simulink library "powerlib_extras"  (Simulink 6.0)
settings: Solver=ode45  SolverMode=SingleTasking  StartTime=0.0  StopTime=10.0  RelTol=1e-3
values from neighbouring files (symbols this model uses):
  Ts = get(handles.edit1,'string')    [powergui.m]
undefined symbols (not defined in the file or in its folder): Ac, Bc, Cc, Dc, Delay_discrete, dend, DiscIntNeverNeededParam, extra_sc, j, numd, test_alpha
libraries: powerlib2 x112, powerlib_extras x70, simulink_extras x25, simulink x12, powerlib_models x8
(part 8 of 9)

== system powerlib_extras/Measurements/3-Phase Sequence Analyzer/PhasorA ==
  in : Inport  Port=1  LatchInput=off
  sin : Inport  Port=2  LatchInput=off
  cos : Inport  Port=3  LatchInput=off
  Gain1 : Gain  Gain=k*f1  SaturateOnIntegerOverflow=on
  Integ2 : Integrator
  Product : Product  SaturateOnIntegerOverflow=on  InputSameDT=on
  Product1 : Product  SaturateOnIntegerOverflow=on  InputSameDT=on
  Real-Imag to Complex : RealImagToComplex
  Sum2 : Sum  Inputs=+-  SaturateOnIntegerOverflow=on  InputSameDT=on
  Sum3 : Sum  Inputs=+-  SaturateOnIntegerOverflow=on  InputSameDT=on
  T : TransportDelay  DelayTime=1/f1
  T1 : TransportDelay  DelayTime=1/f1
  integ1 : Integrator
  Out : Outport  InitialOutput=0
  wires:
  Real-Imag to Complex/1 -> Out/1
  Sum3/1 -> Real-Imag to Complex/2
  Sum2/1 -> Real-Imag to Complex/1
  Product/1 -> integ1/1
  Product1/1 -> Integ2/1
  T/1 -> Sum2/2
  T1/1 -> Sum3/2
  integ1/1 -> T/1, Sum2/1
  Integ2/1 -> T1/1, Sum3/1
  Gain1/1 -> Product1/1, Product/2
  sin/1 -> Product/1
  in/1 -> Gain1/1
  cos/1 -> Product1/2

== system powerlib_extras/Measurements/3-Phase Sequence Analyzer/PhasorB ==
  in : Inport  Port=1  LatchInput=off
  sin : Inport  Port=2  LatchInput=off
  cos : Inport  Port=3  LatchInput=off
  Gain1 : Gain  Gain=k*f1  SaturateOnIntegerOverflow=on
  Integ2 : Integrator
  Product : Product  SaturateOnIntegerOverflow=on  InputSameDT=on
  Product1 : Product  SaturateOnIntegerOverflow=on  InputSameDT=on
  Real-Imag to Complex : RealImagToComplex
  Sum2 : Sum  Inputs=+-  SaturateOnIntegerOverflow=on  InputSameDT=on
  Sum3 : Sum  Inputs=+-  SaturateOnIntegerOverflow=on  InputSameDT=on
  T : TransportDelay  DelayTime=1/f1
  T1 : TransportDelay  DelayTime=1/f1
  integ1 : Integrator
  Out : Outport  InitialOutput=0
  wires:
  cos/1 -> Product1/2
  in/1 -> Gain1/1
  sin/1 -> Product/1
  Gain1/1 -> Product/2, Product1/1
  Integ2/1 -> Sum3/1, T1/1
  integ1/1 -> Sum2/1, T/1
  T1/1 -> Sum3/2
  T/1 -> Sum2/2
  Product1/1 -> Integ2/1
  Product/1 -> integ1/1
  Sum2/1 -> Real-Imag to Complex/1
  Sum3/1 -> Real-Imag to Complex/2
  Real-Imag to Complex/1 -> Out/1

== system powerlib_extras/Measurements/3-Phase Sequence Analyzer/PhasorC ==
  in : Inport  Port=1  LatchInput=off
  sin : Inport  Port=2  LatchInput=off
  cos : Inport  Port=3  LatchInput=off
  Gain1 : Gain  Gain=k*f1  SaturateOnIntegerOverflow=on
  Integ2 : Integrator
  Product : Product  SaturateOnIntegerOverflow=on  InputSameDT=on
  Product1 : Product  SaturateOnIntegerOverflow=on  InputSameDT=on
  Real-Imag to Complex : RealImagToComplex
  Sum2 : Sum  Inputs=+-  SaturateOnIntegerOverflow=on  InputSameDT=on
  Sum3 : Sum  Inputs=+-  SaturateOnIntegerOverflow=on  InputSameDT=on
  T : TransportDelay  DelayTime=1/f1
  T1 : TransportDelay  DelayTime=1/f1
  integ1 : Integrator
  Out : Outport  InitialOutput=0
  wires:
  Real-Imag to Complex/1 -> Out/1
  Sum3/1 -> Real-Imag to Complex/2
  Sum2/1 -> Real-Imag to Complex/1
  Product/1 -> integ1/1
  Product1/1 -> Integ2/1
  T/1 -> Sum2/2
  T1/1 -> Sum3/2
  integ1/1 -> T/1, Sum2/1
  Integ2/1 -> T1/1, Sum3/1
  Gain1/1 -> Product1/1, Product/2
  sin/1 -> Product/1
  in/1 -> Gain1/1
  cos/1 -> Product1/2

== system powerlib_extras/Measurements/3-Phase Sequence Analyzer/Pos. Seq. Computation ==
  In : Inport  Port=1  LatchInput=off
  Enable : EnablePort
  Gain1 : Gain  Gain=[1 a a2]  SaturateOnIntegerOverflow=on
  Gain3 : Gain  Gain=1/3  SaturateOnIntegerOverflow=on
  Sum : Sum  Inputs=1  SaturateOnIntegerOverflow=on  InputSameDT=on
  Out : Outport
  wires:
  Gain1/1 -> Sum/1
  Sum/1 -> Gain3/1
  In/1 -> Gain1/1
  Gain3/1 -> Out/1

== system powerlib_extras/Measurements/3-Phase Sequence Analyzer/Zero Seq. Computation ==
  In : Inport  Port=1  LatchInput=off
  Enable : EnablePort
  Gain3 : Gain  Gain=1/3  SaturateOnIntegerOverflow=on
  Sum : Sum  Inputs=1  SaturateOnIntegerOverflow=on  InputSameDT=on
  Out : Outport
  wires:
  Sum/1 -> Gain3/1
  In/1 -> Sum/1
  Gain3/1 -> Out/1

== system powerlib_extras/Phasor Library/Sequence Analyzer (Phasor Type)/Neg. Seq. Computation ==
  In : Inport  Port=1  LatchInput=off
  Enable : EnablePort
  Gain1 : Gain  Gain=[1 a2 a]  SaturateOnIntegerOverflow=on
  Gain3 : Gain  Gain=1/3  SaturateOnIntegerOverflow=on
  Sum : Sum  Inputs=1  SaturateOnIntegerOverflow=on  InputSameDT=on
  Out : Outport
  wires:
  Gain3/1 -> Out/1
  In/1 -> Gain1/1
  Sum/1 -> Gain3/1
  Gain1/1 -> Sum/1

== system powerlib_extras/Phasor Library/Sequence Analyzer (Phasor Type)/Pos. Seq. Computation ==
  In : Inport  Port=1  LatchInput=off
  Enable : EnablePort
  Gain1 : Gain  Gain=[1 a a2]  SaturateOnIntegerOverflow=on
  Gain3 : Gain  Gain=1/3  SaturateOnIntegerOverflow=on
  Sum : Sum  Inputs=1  SaturateOnIntegerOverflow=on  InputSameDT=on
  Out : Outport
  wires:
  Gain3/1 -> Out/1
  In/1 -> Gain1/1
  Sum/1 -> Gain3/1
  Gain1/1 -> Sum/1

== system powerlib_extras/Phasor Library/Sequence Analyzer (Phasor Type)/Zero Seq. Computation ==
  In : Inport  Port=1  LatchInput=off
  Enable : EnablePort
  Gain3 : Gain  Gain=1/3  SaturateOnIntegerOverflow=on
  Sum : Sum  Inputs=1  SaturateOnIntegerOverflow=on  InputSameDT=on
  Out : Outport
  wires:
  Gain3/1 -> Out/1
  In/1 -> Sum/1
  Sum/1 -> Gain3/1

== system powerlib_extras/Phasor Library/Static Var Compensator (Phasor Type)/Currrent phasor ==
  I1 : Inport  Port=1  LatchInput=off
  I2 : Inport  Port=2  LatchInput=off
  Mux1 : Mux  Inputs=2
  Sum1 : Sum  SaturateOnIntegerOverflow=on  InputSameDT=on
  Sum3 : Sum  SaturateOnIntegerOverflow=on  InputSameDT=on
  a : Gain  Gain=exp(j*2*pi/3)  SaturateOnIntegerOverflow=on
  a^2 : Gain  Gain=exp(-j*2*pi/3)  SaturateOnIntegerOverflow=on
  Ia Ib cmplx : Outport
  wires:
  Mux1/1 -> Ia Ib cmplx/1  "ia ib"
  Sum1/1 -> Mux1/2
  Sum3/1 -> Mux1/1
  a/1 -> Sum1/2
  a^2/1 -> Sum1/1
  I2/1 -> Sum3/2, a/1
  I1/1 -> Sum3/1, a^2/1

== system powerlib_extras/Phasor Library/Static Var Compensator (Phasor Type)/I1 Time delay  Td ==
  I1 cmplx : Inport  Orientation=left  Port=1  LatchInput=off
  Complex to Real-Imag : ComplexToRealImag  Orientation=left
  Real-Imag to Complex : RealImagToComplex  Orientation=left
  Transport Delay1 : TransportDelay  Orientation=left  DelayTime=Td
  Transport Delay2 : TransportDelay  Orientation=left  DelayTime=Td
  Out1 : Outport  Orientation=left
  wires:
  I1 cmplx/1 -> Complex to Real-Imag/1
  Real-Imag to Complex/1 -> Out1/1
  Complex to Real-Imag/1 -> Transport Delay1/1
  Complex to Real-Imag/2 -> Transport Delay2/1
  Transport Delay1/1 -> Real-Imag to Complex/1
  Transport Delay2/1 -> Real-Imag to Complex/2

== system powerlib_extras/Phasor Library/Static Var Compensator (Phasor Type)/I2 Time delay I2 ==
  I1 cmplx : Inport  Orientation=left  Port=1  LatchInput=off
  Complex to Real-Imag : ComplexToRealImag  Orientation=left
  Real-Imag to Complex : RealImagToComplex  Orientation=left
  Transport Delay1 : TransportDelay  Orientation=left  DelayTime=Td
  Transport Delay2 : TransportDelay  Orientation=left  DelayTime=Td
  Out1 : Outport  Orientation=left
  wires:
  Transport Delay2/1 -> Real-Imag to Complex/2
  Transport Delay1/1 -> Real-Imag to Complex/1
  Complex to Real-Imag/2 -> Transport Delay2/1
  Complex to Real-Imag/1 -> Transport Delay1/1
  Real-Imag to Complex/1 -> Out1/1
  I1 cmplx/1 -> Complex to Real-Imag/1

== system powerlib_extras/Phasor Library/Static Var Compensator (Phasor Type)/V1 V2 ==
  Vab Vbc cmplx : Inport  Port=1  LatchInput=off
  (a^2)/3 : Gain  Gain=1/3*exp(-j*2*pi/3)  SaturateOnIntegerOverflow=on
  Demux : Demux  Outputs=2
  Gain : Gain  Gain=1/3  SaturateOnIntegerOverflow=on
  Gain1 : Gain  Gain=1/3  SaturateOnIntegerOverflow=on
  Sum3 : Sum  Inputs=+-  SaturateOnIntegerOverflow=on  InputSameDT=on
  Sum4 : Sum  Inputs=+-  SaturateOnIntegerOverflow=on  InputSameDT=on
  V>pu : Gain  Gain=1/Vbase  SaturateOnIntegerOverflow=on
  a/3 : Gain  Gain=1/3*exp(j*2*pi/3)  SaturateOnIntegerOverflow=on
  V1_pu : Outport
  V2_pu : Outport  Port=2
  wires:
  Sum4/1 -> V2_pu/1  "V2"
  (a^2)/3/1 -> Sum3/2
  Demux/2 -> (a^2)/3/1, a/3/1
  Gain/1 -> Sum3/1
  Vab Vbc cmplx/1 -> V>pu/1
  Gain1/1 -> Sum4/1
  a/3/1 -> Sum4/2
  Demux/1 -> Gain/1, Gain1/1
  Sum3/1 -> V1_pu/1  "V1"
  V>pu/1 -> Demux/1

== system powerlib_extras/Phasor Library/Static Var Compensator (Phasor Type)/Voltage regulator ==
  V1meas (pu) : Inport  Port=1  LatchInput=off
  Vref (pu) : Inport  Port=2  LatchInput=off
  Break algebraic loop : TransferFcn  Orientation=left  Denominator=[100e-6 1]
  Droop : Gain  Orientation=left  Gain=Xs  SaturateOnIntegerOverflow=on
  Integrator : Integrator  LimitOutput=on  UpperSaturationLimit=1  LowerSaturationLimit=-1
  Ki : Gain  Gain=Ki  SaturateOnIntegerOverflow=on
  Product : Product  Orientation=down  SaturateOnIntegerOverflow=on  InputSameDT=on
  Sum : Sum  Inputs=-+-  SaturateOnIntegerOverflow=on  InputSameDT=on
  B (pu) : Outport  InitialOutput=0
  wires:
  Product/1 -> Break algebraic loop/1
  Integrator/1 -> B (pu)/1, Product/2
  Sum/1 -> Ki/1
  Vref (pu)/1 -> Sum/2
  Ki/1 -> Integrator/1
  V1meas (pu)/1 -> Sum/1, Product/1
  Droop/1 -> Sum/3
  Break algebraic loop/1 -> Droop/1

== system powerlib_extras/Control  Blocks/ Synchronized 12-Pulse Generator/12 Flip-Flops/6 Flip-Flop ==
  S : Inport  Port=1  LatchInput=off
  R : Inport  Port=2  LatchInput=off
  Demux : Demux  Outputs=6
  Demux1 : Demux  Outputs=6
  Mux : Mux  Inputs=6
  S-R Flip-Flop{1..6} (6 alike) : simulink_extras/Flip Flops/S-R Flip-Flop  initial_condition=0
  Terminator{,1..5} (6 alike) : Terminator
  Q : Outport
  wires:
  S-R Flip-Flop6/2 -> Terminator5/1
  S-R Flip-Flop5/2 -> Terminator4/1
  S-R Flip-Flop4/2 -> Terminator3/1
  S-R Flip-Flop3/2 -> Terminator2/1
  S-R Flip-Flop2/2 -> Terminator1/1
  S-R Flip-Flop1/1 -> Mux/1
  S-R Flip-Flop2/1 -> Mux/2
  S-R Flip-Flop3/1 -> Mux/3
  S-R Flip-Flop4/1 -> Mux/4
  S-R Flip-Flop5/1 -> Mux/5
  Mux/1 -> Q/1
  S-R Flip-Flop6/1 -> Mux/6
  S-R Flip-Flop1/2 -> Terminator/1
  Demux/1 -> S-R Flip-Flop1/1
  Demux/2 -> S-R Flip-Flop2/1
  Demux/3 -> S-R Flip-Flop3/1
  Demux/4 -> S-R Flip-Flop4/1
  S/1 -> Demux/1
  Demux/6 -> S-R Flip-Flop6/1
  Demux/5 -> S-R Flip-Flop5/1
  R/1 -> Demux1/1
  Demux1/1 -> S-R Flip-Flop1/2
  Demux1/2 -> S-R Flip-Flop2/2
  Demux1/3 -> S-R Flip-Flop3/2
  Demux1/4 -> S-R Flip-Flop4/2
  Demux1/5 -> S-R Flip-Flop5/2
  Demux1/6 -> S-R Flip-Flop6/2

== system powerlib_extras/Control  Blocks/ Synchronized 12-Pulse Generator/12 Flip-Flops/6 Flip-Flop1 ==
  S : Inport  Port=1  LatchInput=off
  R : Inport  Port=2  LatchInput=off
  Demux : Demux  Outputs=6
  Demux1 : Demux  Outputs=6
  Mux : Mux  Inputs=6
  S-R Flip-Flop{1..6} (6 alike) : simulink_extras/Flip Flops/S-R Flip-Flop  initial_condition=0
  Terminator{,1..5} (6 alike) : Terminator
  Q : Outport
  wires:
  Demux1/6 -> S-R Flip-Flop6/2
  Demux1/5 -> S-R Flip-Flop5/2
  Demux1/4 -> S-R Flip-Flop4/2
  Demux1/3 -> S-R Flip-Flop3/2
  Demux1/2 -> S-R Flip-Flop2/2
  Demux1/1 -> S-R Flip-Flop1/2
  R/1 -> Demux1/1
  Demux/5 -> S-R Flip-Flop5/1
  Demux/6 -> S-R Flip-Flop6/1
  S/1 -> Demux/1
  Demux/4 -> S-R Flip-Flop4/1
  Demux/3 -> S-R Flip-Flop3/1
  Demux/2 -> S-R Flip-Flop2/1
  Demux/1 -> S-R Flip-Flop1/1
  S-R Flip-Flop1/2 -> Terminator/1
  S-R Flip-Flop6/1 -> Mux/6
  Mux/1 -> Q/1
  S-R Flip-Flop5/1 -> Mux/5
  S-R Flip-Flop4/1 -> Mux/4
  S-R Flip-Flop3/1 -> Mux/3
  S-R Flip-Flop2/1 -> Mux/2
  S-R Flip-Flop1/1 -> Mux/1
  S-R Flip-Flop2/2 -> Terminator1/1
  S-R Flip-Flop3/2 -> Terminator2/1
  S-R Flip-Flop4/2 -> Terminator3/1
  S-R Flip-Flop5/2 -> Terminator4/1
  S-R Flip-Flop6/2 -> Terminator5/1

== system powerlib_extras/Control  Blocks/Monostable/Edge Detector/NEGATIVE Edge ==
  IN : Inport  Port=1  LatchInput=off
  IN previous : Inport  Port=2  LatchInput=off
  Enable : EnablePort
  Relational Operator1 : RelationalOperator  Operator=>  InputSameDT=on
  OUT : Outport
  wires:
  IN/1 -> Relational Operator1/2
  IN previous/1 -> Relational Operator1/1
  Relational Operator1/1 -> OUT/1

== system powerlib_extras/Control  Blocks/Monostable/Edge Detector/POSITIVE Edge ==
  IN : Inport  Port=1  LatchInput=off
  IN previous : Inport  Port=2  LatchInput=off
  Enable : EnablePort
  Relational Operator1 : RelationalOperator  Operator=>  InputSameDT=on
  OUT : Outport
  wires:
  IN/1 -> Relational Operator1/1
  IN previous/1 -> Relational Operator1/2
  Relational Operator1/1 -> OUT/1

== system powerlib_extras/Discrete  Control Blocks/Discrete Monostable/Edge_Detector/NEGATIVE Edge ==
  IN : Inport  Port=1  LatchInput=off
  IN previous : Inport  Port=2  LatchInput=off
  Enable : EnablePort
  Relational Operator1 : RelationalOperator  Operator=>  InputSameDT=on
  OUT : Outport
  wires:
  IN/1 -> Relational Operator1/2
  IN previous/1 -> Relational Operator1/1
  Relational Operator1/1 -> OUT/1

== system powerlib_extras/Discrete  Control Blocks/Discrete Monostable/Edge_Detector/POSITIVE Edge ==
  IN : Inport  Port=1  LatchInput=off
  IN previous : Inport  Port=2  LatchInput=off
  Enable : EnablePort
  Relational Operator1 : RelationalOperator  Operator=>  InputSameDT=on
  OUT : Outport
  wires:
  IN/1 -> Relational Operator1/1
  IN previous/1 -> Relational Operator1/2
  Relational Operator1/1 -> OUT/1

== system powerlib_extras/Discrete  Control Blocks/Discrete 12-Pulse HVDC Control /Functions (Discrete)/Control Mode ==
  note: CONTROL MODE (#):
      |
      | 0) Blocked
      | 1) Current control
      | 2) Voltage control
      | 3) Alpha minimum limitation
      | 4) Alpha maximum limitation
      | 5) Forced or constant Alpha
  "a_ord_i " : Inport  Port=1  LatchInput=off
  a_ord_v : Inport  Port=2  LatchInput=off
  alpha_ord : Inport  Port=3  LatchInput=off
  Max_i : Inport  Port=4  LatchInput=off
  Min_i : Inport  Port=5  LatchInput=off
  Block : Inport  Port=6  LatchInput=off
  C : Constant  Value=0
  Gain1 : Gain  Gain=3  SaturateOnIntegerOverflow=on
  Gain2 : Gain  Gain=4  SaturateOnIntegerOverflow=on
  Gain3 : Gain  Gain=2  SaturateOnIntegerOverflow=on
  Gain4 : Gain  Gain=5  SaturateOnIntegerOverflow=on
  Logical Operator : Logic
  Logical Operator1 : Logic
  Logical Operator2 : Logic  Inputs=3
  Logical Operator3 : Logic
  Logical Operator4 : Logic  Operator=OR
  Logical Operator5 : Logic  Operator=NOT
  Logical Operator6 : Logic  Operator=NOT
  Logical Operator7 : Logic  Operator=NOT
  Relational Operator : RelationalOperator  Operator=<=  InputSameDT=on
  Relational Operator1 : RelationalOperator  Operator=<=  InputSameDT=on
  Relational Operator2 : RelationalOperator  InputSameDT=on
  Relational Operator3 : RelationalOperator  Operator=>  InputSameDT=on
  Relational Operator4 : RelationalOperator  Operator===  InputSameDT=on
  Sum : Sum  Inputs=+++++  SaturateOnIntegerOverflow=on  InputSameDT=on
  Switch : Switch  Threshold=0.5  SaturateOnIntegerOverflow=on  InputSameDT=on
  mode : Outport
  wires:
  C/1 -> Switch/1
  Sum/1 -> Switch/3
  Switch/1 -> mode/1
  Block/1 -> Switch/2
  "a_ord_i "/1 -> Relational Operator/1, Relational Operator3/1  "a_ord_i"
  a_ord_v/1 -> Relational Operator/2, Relational Operator3/2  "a_ord_v"
  Relational Operator/1 -> Logical Operator3/1  "ACR"
  Logical Operator3/1 -> Sum/1
  Gain3/1 -> Sum/2
  Relational Operator3/1 -> Logical Operator/1  "AVR"
  Logical Operator/1 -> Gain3/1
  alpha_ord/1 -> Relational Operator1/1, Relational Operator2/1  "alpha_ord"
  Relational Operator1/1 -> Logical Operator4/1, Logical Operator6/1, Logical Operator1/1  "AMIN"
  Logical Operator4/1 -> Logical Operator5/1
  Relational Operator2/1 -> Logical Operator4/2, Logical Operator2/2  "AMAX"
  Logical Operator6/1 -> Logical Operator2/1
  Logical Operator2/1 -> Gain2/1
  Gain1/1 -> Sum/3
  Gain2/1 -> Sum/4
  Min_i/1 -> Relational Operator1/2, Relational Operator4/1
  Max_i/1 -> Relational Operator2/2, Relational Operator4/2
  Relational Operator4/1 -> Gain4/1  "AFOR"
  Logical Operator1/1 -> Gain1/1
  Gain4/1 -> Sum/5, Logical Operator7/1
  Logical Operator7/1 -> Logical Operator1/2, Logical Operator2/3
  Logical Operator5/1 -> Logical Operator/2, Logical Operator3/2

== system powerlib_extras/Discrete  Control Blocks/Discrete 12-Pulse HVDC Control /Functions (Discrete)/Current Regulator ==
  note: PI Regulator With external limits (Linearized Kp) (Discrete)
  Max_i : Inport  Port=1  LatchInput=off
  Min_i : Inport  Port=2  LatchInput=off
  ERR : Inport  Port=3  LatchInput=off
  Max_pi : Inport  Port=4  LatchInput=off
  Min_pi : Inport  Port=5  LatchInput=off
  Alpha_lin : Inport  Port=6  LatchInput=off
  Max_lin : Inport  Port=7  LatchInput=off
  Min_lin : Inport  Port=8  LatchInput=off
  Inv : Inport  Port=9  LatchInput=off
  Ground : Ground
  KI (deg per pu per s) : Gain  Gain=Ki  SaturateOnIntegerOverflow=on
  Kp (deg per pu) : Constant  Value=Kp
  Kp Linearisation : Subsystem
  Prod : Product  SaturateOnIntegerOverflow=on  InputSameDT=on
  S16 : Subsystem  mask(Integrator  With  External  Dynamic  Limits (Discrete)){k=1, ic=IC_i, st=pas}
      mask prompts: k "Gain:"; ic "Initial Condition:"; st "Sample time: (s)"
      mask Display: disp('Integrator\nwith\nExternal Limits\nGain & Reset & Hold\n(Discrete)')
  S6 : Subsystem
      mask Type: Limiter with External Limits
      mask Display: disp('      Limiter\n')
  Sum : Sum  SaturateOnIntegerOverflow=on  InputSameDT=on
  Alpha_ord : Outport  InitialOutput=0
  wires:
  Alpha_lin/1 -> Kp Linearisation/1(Alpha_lin)
  S6/1("  ") -> Alpha_ord/1
  Kp Linearisation/1(Kp_lin) -> Prod/1
  Kp (deg per pu)/1 -> Kp Linearisation/2(Kp)
  KI (deg per pu per s)/1 -> S16/3(In)
  Max_i/1 -> S16/1(Max)
  Min_i/1 -> S16/2(Min)
  Sum/1 -> S6/2(In)
  Max_pi/1 -> S6/1(MAX)
  Min_pi/1 -> S6/3(MIN)
  S16/1(Out) -> Sum/2
  ERR/1 -> KI (deg per pu per s)/1, Prod/2
  Ground/1 -> S16/4(Reset), S16/5(Hold), S16/6(Reset Value)
  Inv/1 -> Kp Linearisation/3(Inv)
  Max_lin/1 -> Kp Linearisation/5(Max_lin)
  Min_lin/1 -> Kp Linearisation/4(Min_lin)
  Prod/1 -> Sum/1

== system powerlib_extras/Discrete  Control Blocks/Discrete 12-Pulse HVDC Control /Functions (Discrete)/Filtre passe-bas 1er ordre  (DISCRET)3 ==
  In : Inport  Port=1  LatchInput=off
  Discrete Transfer Fcn : DiscreteTransferFcn  Numerator=numd  Denominator=dend  SampleTime=Pas
  Out : Outport  InitialOutput=0
  wires:
  Discrete Transfer Fcn/1 -> Out/1
  In/1 -> Discrete Transfer Fcn/1

== system powerlib_extras/Discrete  Control Blocks/Discrete 12-Pulse HVDC Control /Functions (Discrete)/Filtre passe-bas 1er ordre  (DISCRET)4 ==
  In : Inport  Port=1  LatchInput=off
  Discrete Transfer Fcn : DiscreteTransferFcn  Numerator=numd  Denominator=dend  SampleTime=Pas
  Out : Outport  InitialOutput=0
  wires:
  In/1 -> Discrete Transfer Fcn/1
  Discrete Transfer Fcn/1 -> Out/1

== system powerlib_extras/Discrete  Control Blocks/Discrete 12-Pulse HVDC Control /Functions (Discrete)/Filtre passe-bas 1er ordre  (DISCRET)5 ==
  In : Inport  Port=1  LatchInput=off
  Discrete Transfer Fcn : DiscreteTransferFcn  Numerator=numd  Denominator=dend  SampleTime=Pas
  Out : Outport  InitialOutput=0
  wires:
  Discrete Transfer Fcn/1 -> Out/1
  In/1 -> Discrete Transfer Fcn/1

== system powerlib_extras/Discrete  Control Blocks/Discrete 12-Pulse HVDC Control /Functions (Discrete)/Filtre passe-bas 1er ordre  (DISCRET)6 ==
  In : Inport  Port=1  LatchInput=off
  Discrete Transfer Fcn : DiscreteTransferFcn  Numerator=numd  Denominator=dend  SampleTime=Pas
  Out : Outport  InitialOutput=0
  wires:
  Discrete Transfer Fcn/1 -> Out/1
  In/1 -> Discrete Transfer Fcn/1

== system powerlib_extras/Discrete  Control Blocks/Discrete 12-Pulse HVDC Control /Functions (Discrete)/S6 ==
  note: Limiter
      | with external
      | limits
  MAX : Inport  Port=1  LatchInput=off
  In : Inport  Port=2  LatchInput=off
  MIN : Inport  Port=3  LatchInput=off
  MinMax : MinMax  Function=max  Inputs=2  SaturateOnIntegerOverflow=on  InputSameDT=on
  MinMax1 : MinMax  Inputs=2  SaturateOnIntegerOverflow=on  InputSameDT=on
  "  " : Outport  InitialOutput=0
  wires:
  In/1 -> MinMax1/2
  MinMax/1 -> "  "/1
  MIN/1 -> MinMax/1
  MAX/1 -> MinMax1/1
  MinMax1/1 -> MinMax/2

== system powerlib_extras/Discrete  Control Blocks/Discrete 12-Pulse HVDC Control /Functions (Discrete)/VDCOL ==
  note: Voltage Dependant Current Order Limiter (VDCOL) (Discrete)
  Id_ref (pu) : Inport  Port=1  LatchInput=off
  Vd (pu) : Inport  Port=2  LatchInput=off
  Constant : Constant  Value=Id_min
  Constant1 : Constant  Value=Vd_min
  Constant2 : Constant  Value=Vd_seuil
  Constant3 : Constant
  Constant4 : Constant
  Constant5 : Constant  Value=Tu
  Logical Operator : Logic  Orientation=left  Operator=NOT
  Math Function : Math  Operator=reciprocal  SaturateOnIntegerOverflow=on
  Max = 10 Min=Id_min_abs : Saturate  UpperLimit=10  LowerLimit=Id_min_abs
  MinMax2 : MinMax  Function=max  Inputs=2  SaturateOnIntegerOverflow=on  InputSameDT=on
  MinMax3 : MinMax  Inputs=2  SaturateOnIntegerOverflow=on  InputSameDT=on
  PB_R : Subsystem  mask(Low Pass Filter With Reset (discrete: Zoh method, Forward Euler)){ic=1, dt=pas}
      mask prompts: ic "Initial condition:"; dt "Sample time (s)"
      mask help:
      | The output will be reset to the input value (Time constant = 0)  during the input (2) is True. The Time constant (T) is defined by
      | input (3).
      mask Display:
      | plot(0,0,100,100,[90,80,70,60,50,40,29,20,10],[60,55,52,55,60,65,67,65,60],[89,80,71,60,50,40,30,20,10],[40,35,32,35,40,45,47,45,40],[56,44],[70,50]);
      | disp('\n\nD')
  Product{,1..4} (5 alike) : Product  SaturateOnIntegerOverflow=on  InputSameDT=on
  Relational Operator : RelationalOperator  InputSameDT=on
  Sum : Sum  Inputs=+-  SaturateOnIntegerOverflow=on  InputSameDT=on
  Sum1 : Sum  Inputs=+-  SaturateOnIntegerOverflow=on  InputSameDT=on
  Sum2 : Sum  Inputs=+-  SaturateOnIntegerOverflow=on  InputSameDT=on
  Sum3 : Sum  SaturateOnIntegerOverflow=on  InputSameDT=on
  Unit Delay : UnitDelay  Orientation=left  SampleTime=pas
  Id_ref_lim : Outport  InitialOutput=0
  Vd_filt : Outport  Port=2  InitialOutput=0
  wires:
  Relational Operator/1 -> Unit Delay/1
  Max = 10 Min=Id_min_abs/1 -> MinMax2/2
  MinMax2/1 -> MinMax3/2
  Product1/1 -> MinMax2/1  "Idref_lim"
  Constant2/1 -> Product3/1, Sum1/1
  Product/1 -> Product3/2, Product2/1  "A"
  Product3/1 -> Sum2/2
  MinMax3/1 -> Id_ref_lim/1
  Id_ref (pu)/1 -> Product4/2, MinMax3/1, Product1/1
  Product4/1 -> Max = 10 Min=Id_min_abs/1  "min"
  Constant/1 -> Product4/1, Sum/2
  Sum3/1 -> Product1/2
  Product2/1 -> Sum3/2
  Sum2/1 -> Sum3/1  "B"
  Constant4/1 -> Sum2/1
  Math Function/1 -> Product/2
  Sum/1 -> Product/1
  Sum1/1 -> Math Function/1
  Constant1/1 -> Sum1/2
  Constant3/1 -> Sum/1
  Constant5/1 -> PB_R/3(T)
  PB_R/1(Out) -> Product2/2, Vd_filt/1, Relational Operator/2
  Vd (pu)/1 -> PB_R/1("In "), Relational Operator/1
  Unit Delay/1 -> Logical Operator/1
  Logical Operator/1 -> PB_R/2(Reset)

== system powerlib_extras/Discrete  Control Blocks/Discrete 12-Pulse HVDC Control /Functions (Discrete)/Voltage Regulator ==
  note: PI Regulator With external limits (Linearized Kp) (Discrete)
  Max_i : Inport  Port=1  LatchInput=off
  Min_i : Inport  Port=2  LatchInput=off
  ERR : Inport  Port=3  LatchInput=off
  Max_pi : Inport  Port=4  LatchInput=off
  Min_pi : Inport  Port=5  LatchInput=off
  Alpha_lin : Inport  Port=6  LatchInput=off
  Max_lin : Inport  Port=7  LatchInput=off
  Min_lin : Inport  Port=8  LatchInput=off
  Inv : Inport  Port=9  LatchInput=off
  Ground : Ground
  KI (deg per pu per s) : Gain  Gain=Ki  SaturateOnIntegerOverflow=on
  Kp (deg per pu) : Constant  Value=Kp
  Kp Linearisation : Subsystem
  Prod : Product  SaturateOnIntegerOverflow=on  InputSameDT=on
  S16 : Subsystem  mask(Integrator  With  External  Dynamic  Limits (Discrete)){k=1, ic=IC_i, st=pas}
      mask prompts: k "Gain:"; ic "Initial Condition:"; st "Sample time: (s)"
      mask Display: disp('Integrator\nwith\nExternal Limits\nGain & Reset & Hold\n(Discrete)')
  S6 : Subsystem
      mask Type: Limiter with External Limits
      mask Display: disp('      Limiter\n')
  Sum : Sum  SaturateOnIntegerOverflow=on  InputSameDT=on
  Alpha_ord : Outport  InitialOutput=0
  wires:
  Prod/1 -> Sum/1
  Min_lin/1 -> Kp Linearisation/4(Min_lin)
  Max_lin/1 -> Kp Linearisation/5(Max_lin)
  Inv/1 -> Kp Linearisation/3(Inv)
  Ground/1 -> S16/6(Reset Value), S16/5(Hold), S16/4(Reset)
  ERR/1 -> Prod/2, KI (deg per pu per s)/1
  S16/1(Out) -> Sum/2
  Min_pi/1 -> S6/3(MIN)
  Max_pi/1 -> S6/1(MAX)
  Sum/1 -> S6/2(In)
  Min_i/1 -> S16/2(Min)
  Max_i/1 -> S16/1(Max)
  KI (deg per pu per s)/1 -> S16/3(In)
  Kp (deg per pu)/1 -> Kp Linearisation/2(Kp)
  Kp Linearisation/1(Kp_lin) -> Prod/1
  S6/1("  ") -> Alpha_ord/1
  Alpha_lin/1 -> Kp Linearisation/1(Alpha_lin)

== system powerlib_extras/Discrete  Control Blocks/Discrete 12-Pulse HVDC Control /Functions (Discrete)/alpha_init ==
  In1 : Inport  Port=1  PortDimensions=1  LatchInput=off
  IC : InitialCondition  Value=min(ICi_V,ICi_I)
  Out1 : Outport
  wires:
  IC/1 -> Out1/1
  In1/1 -> IC/1

== system powerlib_extras/Discrete  Control Blocks/Discrete 3-phase PWM Generator/2-level Type/Carriers Generator ==
  theta : Inport  Port=1  LatchInput=off
  Gain1 : Gain  Gain=2/pi  SaturateOnIntegerOverflow=on
  Trigonometric Function : Trigonometry  Operator=asin
  Trigonometric Function3 : Trigonometry
  C : Outport
  wires:
  Gain1/1 -> C/1  "Carrier"
  theta/1 -> Trigonometric Function3/1
  Trigonometric Function3/1 -> Trigonometric Function/1
  Trigonometric Function/1 -> Gain1/1

== system powerlib_extras/Discrete  Control Blocks/Discrete 3-phase PWM Generator/3-level Type/Carriers Generator ==
  theta : Inport  Port=1  LatchInput=off
  Constant2 : Constant  Value=0.5
  Gain1 : Gain  Gain=1/pi  SaturateOnIntegerOverflow=on
  Sum1 : Sum  SaturateOnIntegerOverflow=on  InputSameDT=on
  Sum2 : Sum  Inputs=+-  SaturateOnIntegerOverflow=on  InputSameDT=on
  Trigonometric Function : Trigonometry  Operator=asin
  Trigonometric Function3 : Trigonometry
  C+ : Outport
  C- : Outport  Port=2
  wires:
  Trigonometric Function/1 -> Gain1/1
  Trigonometric Function3/1 -> Trigonometric Function/1
  Gain1/1 -> Sum1/1, Sum2/1
  Constant2/1 -> Sum2/2, Sum1/2
  Sum2/1 -> C-/1  "Carrier 1-"
  Sum1/1 -> C+/1  "Carrier 1+"
  theta/1 -> Trigonometric Function3/1

== system powerlib_extras/Discrete  Control Blocks/Discrete 3-phase PWM Generator/3-level Type/State-to-Pulses Decoder ==
  note: + Vdc --------------------------
  note: - Vdc--------------------------
  note: N -----------
  note: |
      | |
      | |
      | |
      | |
      | |
      | |
      | |
      | |
      | |
      | |
  note: ---------- A
  note: ----------[D]---------
  note: ----------[D]---------
  note: |
      | |
      | [Q4]
      | |
      | |
      | |
  note: |
      | |
      | [Q3]
      | |
      | |
  note: |
      | |
      | [Q2]
      | |
      | |
  note: |
      | |
      | |
      | [Q1]
      | |
      | |
  note: Phase C: 9 to 12
  note: Phase A: 1 to 4
  note: Phase B: 5 to 8
  note: 3-phase State-to-Pulses Decoder
  note: --------------------------------------------------------------
  note: |
      | |
      | |
      | |
      | |
      | |
      | |
      | |
      | |
  note: 1
  note: 1
  note: 0
  note: 0
  note: -1
  note: 0
  note: 1
  note: 1
  note: 0
  note: 0
  note: Q4
  note: Q3
  note: Q2
  note: Q1
  note: 0
  note: 0
  note: 1
  note: 1
  note: Firing pulses
  note: 1
  note: State
  State : Inport  Port=1  PortDimensions=3  LatchInput=off
  Constant11 : Constant  Value=[1 1 0 0]
  Constant12 : Constant  Value=[0 0 1 1]
  Constant13 : Constant  Value=[0 1 1 0]
  Constant2 : Constant  Value=2
  Demux : Demux  Outputs=3
  Multiport Switch : MultiPortSwitch  Inputs=3  InputSameDT=on
  Multiport Switch3 : MultiPortSwitch  Inputs=3  InputSameDT=on
  Multiport Switch4 : MultiPortSwitch  Inputs=3  InputSameDT=on
  Mux : Mux  Inputs=[4 4 4]
  Sum : Sum  SaturateOnIntegerOverflow=on  InputSameDT=on
  Pulses : Outport
  wires:
  Multiport Switch4/1 -> Mux/3
  Multiport Switch3/1 -> Mux/2
  Multiport Switch/1 -> Mux/1
  Constant11/1 -> Multiport Switch4/4, Multiport Switch3/4, Multiport Switch/4
  Constant13/1 -> Multiport Switch4/3, Multiport Switch3/3, Multiport Switch/3
  Constant12/1 -> Multiport Switch4/2, Multiport Switch3/2, Multiport Switch/2
  Demux/3 -> Multiport Switch4/1
  Demux/2 -> Multiport Switch3/1
  Demux/1 -> Multiport Switch/1
  Constant2/1 -> Sum/2
  State/1 -> Sum/1
  Sum/1 -> Demux/1
  Mux/1 -> Pulses/1

== system powerlib_extras/Discrete  Control Blocks/Discrete 3-phase PWM Generator/3-level Type/State-to-Pulses Decoder1 ==
  note: State
  note: 1
  note: Firing pulses
  note: 1
  note: 1
  note: 0
  note: 0
  note: Q1
  note: Q2
  note: Q3
  note: Q4
  note: 0
  note: 0
  note: 1
  note: 1
  note: 0
  note: -1
  note: 0
  note: 0
  note: 1
  note: 1
  note: |
      | |
      | |
      | |
      | |
      | |
      | |
      | |
      | |
  note: --------------------------------------------------------------
  note: 3-phase State-to-Pulses Decoder
  note: Phase B: 5 to 8
  note: Phase A: 1 to 4
  note: Phase C: 9 to 12
  note: |
      | |
      | |
      | [Q1]
      | |
      | |
  note: |
      | |
      | [Q2]
      | |
      | |
  note: |
      | |
      | [Q3]
      | |
      | |
  note: |
      | |
      | [Q4]
      | |
      | |
      | |
  note: ----------[D]---------
  note: ----------[D]---------
  note: ---------- A
  note: |
      | |
      | |
      | |
      | |
      | |
      | |
      | |
      | |
      | |
      | |
  note: N -----------
  note: - Vdc--------------------------
  note: + Vdc --------------------------
  State : Inport  Port=1  PortDimensions=3  LatchInput=off
  Constant11 : Constant  Value=[1 1 0 0]
  Constant12 : Constant  Value=[0 0 1 1]
  Constant13 : Constant  Value=[0 1 1 0]
  Constant2 : Constant  Value=2
  Demux : Demux  Outputs=3
  Multiport Switch : MultiPortSwitch  Inputs=3  InputSameDT=on
  Multiport Switch3 : MultiPortSwitch  Inputs=3  InputSameDT=on
  Multiport Switch4 : MultiPortSwitch  Inputs=3  InputSameDT=on
  Mux : Mux  Inputs=[4 4 4]
  Sum : Sum  SaturateOnIntegerOverflow=on  InputSameDT=on
  Pulses : Outport
  wires:
  Mux/1 -> Pulses/1
  Sum/1 -> Demux/1
  State/1 -> Sum/1
  Constant2/1 -> Sum/2
  Demux/1 -> Multiport Switch/1
  Demux/2 -> Multiport Switch3/1
  Demux/3 -> Multiport Switch4/1
  Constant12/1 -> Multiport Switch/2, Multiport Switch3/2, Multiport Switch4/2
  Constant13/1 -> Multiport Switch/3, Multiport Switch3/3, Multiport Switch4/3
  Constant11/1 -> Multiport Switch/4, Multiport Switch3/4, Multiport Switch4/4
  Multiport Switch/1 -> Mux/1
  Multiport Switch3/1 -> Mux/2
  Multiport Switch4/1 -> Mux/3

== system powerlib_extras/Discrete  Control Blocks/Discrete HVDC Controller/Current Regulator/Kp Linearisation ==
  note: Kp Linearization
  Alpha_lin : Inport  Port=1  LatchInput=off
  Kp : Inport  Port=2  LatchInput=off
  Inv : Inport  Port=3  LatchInput=off
  Min_lin : Inport  Port=4  LatchInput=off
  Max_lin : Inport  Port=5  LatchInput=off
  Constant3 : Constant  Value=On_lin
  Data Type  Conversion : DataTypeConversion  OutDataTypeMode=boolean  SaturateOnIntegerOverflow=on  RndMeth=Zero
  Logical Operator : Logic  Operator=NOT
  Logical Operator1 : Logic  Operator=NOT
  Math Function : Math  Operator=reciprocal  SaturateOnIntegerOverflow=on
  Prod2 : Product  Inputs=3  SaturateOnIntegerOverflow=on  InputSameDT=on
  S6 : Subsystem
      mask Type: Limiter with External Limits
      mask Display: disp('      Limiter\n')
  Switch : Switch  Threshold=0.5  SaturateOnIntegerOverflow=on  InputSameDT=on
  Switch1 : Switch  Threshold=0.5  SaturateOnIntegerOverflow=on  InputSameDT=on
  Trigonometric Function : Trigonometry
  Trigonometric Function1 : Trigonometry
  k : Gain  Gain=pi/180  SaturateOnIntegerOverflow=on
  k1 : Gain  Gain=pi/180  SaturateOnIntegerOverflow=on
  Kp_lin : Outport  InitialOutput=0
  wires:
  Data Type  Conversion/1 -> Logical Operator1/1
  Constant3/1 -> Data Type  Conversion/1
  Min_lin/1 -> S6/3(MIN), Switch/1
  Max_lin/1 -> S6/1(MAX), Switch/3
  Alpha_lin/1 -> S6/2(In)
  Math Function/1 -> Prod2/2
  Trigonometric Function1/1 -> Math Function/1
  k/1 -> Trigonometric Function1/1
  Kp/1 -> Prod2/3, Switch1/1
  Inv/1 -> Logical Operator/1
  Logical Operator/1 -> Switch/2
  Trigonometric Function/1 -> Prod2/1
  S6/1("  ") -> k/1
  k1/1 -> Trigonometric Function/1
  Switch/1 -> k1/1
  Switch1/1 -> Kp_lin/1
  Prod2/1 -> Switch1/3
  Logical Operator1/1 -> Switch1/2  "Off"

== system powerlib_extras/Discrete  Control Blocks/Discrete HVDC Controller/Current Regulator/S16 ==
  note: INTEGRATOR with External limits & Reset & Hold
  note: Gain * dt
  Max : Inport  Port=1  LatchInput=off
  Min : Inport  Port=2  LatchInput=off
  In : Inport  Port=3  LatchInput=off
  Reset : Inport  Port=4  LatchInput=off
  Hold : Inport  Port=5  LatchInput=off
  Reset Value : Inport  Port=6  LatchInput=off
  Gain1 : Gain  Gain=k*dt  SaturateOnIntegerOverflow=on
  IC = ic : UnitDelay  X0=ic  SampleTime=dt
  Logical Operator4 : Logic  Operator=OR
  MinMax : MinMax  Inputs=2  SaturateOnIntegerOverflow=on  InputSameDT=on
  MinMax1 : MinMax  Function=max  Inputs=2  SaturateOnIntegerOverflow=on  InputSameDT=on
  S6 : Subsystem
      mask Type: Limiter with External Limits
      mask Display: disp('      Limiter\n')
  Sum : Sum  SaturateOnIntegerOverflow=on  InputSameDT=on
  Switch2 : Switch  Threshold=0.5  SaturateOnIntegerOverflow=on  InputSameDT=on
  Switch3 : Switch  Threshold=0.5  SaturateOnIntegerOverflow=on  InputSameDT=on
  Switch7 : Switch  Threshold=0.5  SaturateOnIntegerOverflow=on  InputSameDT=on
  Out : Outport  InitialOutput=0
  wires:
  Gain1/1 -> Sum/1
  In/1 -> Gain1/1
  Sum/1 -> S6/2(In)
  S6/1("  ") -> Out/1, IC = ic/1
  Hold/1 -> Logical Operator4/1
  Reset/1 -> Switch7/2, Logical Operator4/2
  Logical Operator4/1 -> Switch2/2, Switch3/2
  Switch2/1 -> MinMax/1
  Max/1 -> Switch2/3, MinMax/2
  Reset Value/1 -> Switch7/1
  MinMax/1 -> S6/1(MAX)
  MinMax1/1 -> S6/3(MIN)
  Switch3/1 -> MinMax1/1
  Min/1 -> Switch3/3, MinMax1/2
  IC = ic/1 -> Switch7/3
  Switch7/1 -> Switch2/1, Sum/2, Switch3/1

== system powerlib_extras/Discrete  Control Blocks/Discrete HVDC Controller/Current Regulator/S6 ==
  note: Limiter
      | with external
      | limits
  MAX : Inport  Port=1  LatchInput=off
  In : Inport  Port=2  LatchInput=off
  MIN : Inport  Port=3  LatchInput=off
  MinMax : MinMax  Function=max  Inputs=2  SaturateOnIntegerOverflow=on  InputSameDT=on
  MinMax1 : MinMax  Inputs=2  SaturateOnIntegerOverflow=on  InputSameDT=on
  "  " : Outport  InitialOutput=0
  wires:
  In/1 -> MinMax1/2
  MinMax/1 -> "  "/1
  MIN/1 -> MinMax/1
  MAX/1 -> MinMax1/1
  MinMax1/1 -> MinMax/2

== system powerlib_extras/Discrete  Control Blocks/Discrete HVDC Controller/Gamma Error/S6 ==
  note: Limiter
      | with external
      | limits
  MAX : Inport  Port=1  LatchInput=off
  In : Inport  Port=2  LatchInput=off
  MIN : Inport  Port=3  LatchInput=off
  MinMax : MinMax  Function=max  Inputs=2  SaturateOnIntegerOverflow=on  InputSameDT=on
  MinMax1 : MinMax  Inputs=2  SaturateOnIntegerOverflow=on  InputSameDT=on
  "  " : Outport  InitialOutput=0
  wires:
  MinMax1/1 -> MinMax/2
  MAX/1 -> MinMax1/1
  MIN/1 -> MinMax/1
  MinMax/1 -> "  "/1
  In/1 -> MinMax1/2

== system powerlib_extras/Discrete  Control Blocks/Discrete HVDC Controller/Gamma Regulator/Gamma Regulator ==
  note: PI Regulator With external limits (Linearized Kp) (Discrete)
  Max_i : Inport  Port=1  LatchInput=off
  Min_i : Inport  Port=2  LatchInput=off
  ERR : Inport  Port=3  LatchInput=off
  Max_pi : Inport  Port=4  LatchInput=off
  Min_pi : Inport  Port=5  LatchInput=off
  Alpha_lin : Inport  Port=6  LatchInput=off
  Max_lin : Inport  Port=7  LatchInput=off
  Min_lin : Inport  Port=8  LatchInput=off
  Inv : Inport  Port=9  LatchInput=off
  Ground : Ground
  KI (deg per pu per s) : Gain  Gain=Ki  SaturateOnIntegerOverflow=on
  Kp (deg per pu) : Constant  Value=Kp
  Kp Linearisation : Subsystem
  Prod : Product  SaturateOnIntegerOverflow=on  InputSameDT=on
  S16 : Subsystem  mask(Integrator  With  External  Dynamic  Limits (Discrete)){k=1, ic=IC_i, st=pas}
      mask prompts: k "Gain:"; ic "Initial Condition:"; st "Sample time: (s)"
      mask Display: disp('Integrator\nwith\nExternal Limits\nGain & Reset & Hold\n(Discrete)')
  S6 : Subsystem
      mask Type: Limiter with External Limits
      mask Display: disp('      Limiter\n')
  Sum : Sum  SaturateOnIntegerOverflow=on  InputSameDT=on
  Alpha_ord : Outport  InitialOutput=0
  wires:
  Alpha_lin/1 -> Kp Linearisation/1(Alpha_lin)
  S6/1("  ") -> Alpha_ord/1
  Kp Linearisation/1(Kp_lin) -> Prod/1
  Kp (deg per pu)/1 -> Kp Linearisation/2(Kp)
  KI (deg per pu per s)/1 -> S16/3(In)
  Max_i/1 -> S16/1(Max)
  Min_i/1 -> S16/2(Min)
  Sum/1 -> S6/2(In)
  Max_pi/1 -> S6/1(MAX)
  Min_pi/1 -> S6/3(MIN)
  S16/1(Out) -> Sum/2
  ERR/1 -> KI (deg per pu per s)/1, Prod/2
  Ground/1 -> S16/4(Reset), S16/5(Hold), S16/6(Reset Value)
  Inv/1 -> Kp Linearisation/3(Inv)
  Max_lin/1 -> Kp Linearisation/5(Max_lin)
  Min_lin/1 -> Kp Linearisation/4(Min_lin)
  Prod/1 -> Sum/1

== system powerlib_extras/Discrete  Control Blocks/Discrete HVDC Controller/Voltage Dependant Current Order Limiter/PB_R ==
  note: Silvano Casoria
      | Laboratoire simulation de reseaux, IREQ
  note: LOW PASS Filter & RESET
      | (Zoh methode)
  "In " : Inport  Port=1  LatchInput=off
  Reset : Inport  Port=2  LatchInput=off
  T : Inport  Port=3  LatchInput=off
  Constant : Constant  Value=dt
  IC= ic : UnitDelay  Orientation=left  X0=ic  SampleTime=dt
  Math Function : Math  Operator=reciprocal  SaturateOnIntegerOverflow=on
  Product : Product  Inputs=3  SaturateOnIntegerOverflow=on  InputSameDT=on
  Sum : Sum  Inputs=+-  SaturateOnIntegerOverflow=on  InputSameDT=on
  Sum1 : Sum  SaturateOnIntegerOverflow=on  InputSameDT=on
  Switch : Switch  Threshold=0.5  SaturateOnIntegerOverflow=on  InputSameDT=on
  Out : Outport  InitialOutput=0
  wires:
  IC= ic/1 -> Sum/2, Sum1/2
  "In "/1 -> Sum/1, Switch/1
  Reset/1 -> Switch/2
  Sum1/1 -> Out/1, Switch/3
  Switch/1 -> IC= ic/1
  Product/1 -> Sum1/1
  Sum/1 -> Product/2
  Math Function/1 -> Product/1
  T/1 -> Math Function/1
  Constant/1 -> Product/3

== system powerlib_extras/Discrete  Control Blocks/Discrete HVDC Controller/Voltage Error/S6 ==
  note: Limiter
      | with external
      | limits
  MAX : Inport  Port=1  LatchInput=off
  In : Inport  Port=2  LatchInput=off
  MIN : Inport  Port=3  LatchInput=off
  MinMax : MinMax  Function=max  Inputs=2  SaturateOnIntegerOverflow=on  InputSameDT=on
  MinMax1 : MinMax  Inputs=2  SaturateOnIntegerOverflow=on  InputSameDT=on
  "  " : Outport  InitialOutput=0
  wires:
  In/1 -> MinMax1/2
  MinMax/1 -> "  "/1
  MIN/1 -> MinMax/1
  MAX/1 -> MinMax1/1
  MinMax1/1 -> MinMax/2

== system powerlib_extras/Discrete  Control Blocks/Discrete HVDC Controller/Voltage Regulator/Voltage Regulator ==
  note: PI Regulator With external limits (Linearized Kp) (Discrete)
  Max_i : Inport  Port=1  LatchInput=off
  Min_i : Inport  Port=2  LatchInput=off
  ERR : Inport  Port=3  LatchInput=off
  Max_pi : Inport  Port=4  LatchInput=off
  Min_pi : Inport  Port=5  LatchInput=off
  Alpha_lin : Inport  Port=6  LatchInput=off
  Max_lin : Inport  Port=7  LatchInput=off
  Min_lin : Inport  Port=8  LatchInput=off
  Inv : Inport  Port=9  LatchInput=off
  Ground : Ground
  KI (deg per pu per s) : Gain  Gain=Ki  SaturateOnIntegerOverflow=on
  Kp (deg per pu) : Constant  Value=Kp
  Kp Linearisation : Subsystem
  Prod : Product  SaturateOnIntegerOverflow=on  InputSameDT=on
  S16 : Subsystem  mask(Integrator  With  External  Dynamic  Limits (Discrete)){k=1, ic=IC_i, st=pas}
      mask prompts: k "Gain:"; ic "Initial Condition:"; st "Sample time: (s)"
      mask Display: disp('Integrator\nwith\nExternal Limits\nGain & Reset & Hold\n(Discrete)')
  S6 : Subsystem
      mask Type: Limiter with External Limits
      mask Display: disp('      Limiter\n')
  Sum : Sum  SaturateOnIntegerOverflow=on  InputSameDT=on
  Alpha_ord : Outport  InitialOutput=0
  wires:
  Prod/1 -> Sum/1
  Min_lin/1 -> Kp Linearisation/4(Min_lin)
  Max_lin/1 -> Kp Linearisation/5(Max_lin)
  Inv/1 -> Kp Linearisation/3(Inv)
  Ground/1 -> S16/6(Reset Value), S16/5(Hold), S16/4(Reset)
  ERR/1 -> Prod/2, KI (deg per pu per s)/1
  S16/1(Out) -> Sum/2
  Min_pi/1 -> S6/3(MIN)
  Max_pi/1 -> S6/1(MAX)
  Sum/1 -> S6/2(In)
  Min_i/1 -> S16/2(Min)
  Max_i/1 -> S16/1(Max)
  KI (deg per pu per s)/1 -> S16/3(In)
  Kp (deg per pu)/1 -> Kp Linearisation/2(Kp)
  Kp Linearisation/1(Kp_lin) -> Prod/1
  S6/1("  ") -> Alpha_ord/1
  Alpha_lin/1 -> Kp Linearisation/1(Alpha_lin)

== system powerlib_extras/Discrete  Control Blocks/Discrete SV PWM Generator/SV Modulator Pattern #1/Compute time duration of switching states (Ta,Tb,To)  ==
  note: TaTbTo
  note: To=(1/Fc-Ta-Tb)
  note: Tb=m*sin(alpha1) * (1/Fc)
  note: Ta=m*cos(alpha1+30)* (1/Fc)
  alpha : Inport  Port=1  LatchInput=off
  m : Inport  Port=2  LatchInput=off
  Sn : Inport  Port=3  LatchInput=off
  Odd_S : Inport  Port=4  LatchInput=off
  1/Fc : Gain  Gain=1/Fc  SaturateOnIntegerOverflow=on
  Constant : Constant  Value=pi/6
  Constant1 : Constant  Value=pi/3
  Constant2 : Constant
  Constant8 : Constant
  Mux : Mux  Inputs=2
  Mux1 : Mux  Inputs=2
  Product : Product  SaturateOnIntegerOverflow=on
  Product1 : Product  SaturateOnIntegerOverflow=on
  Selector1 : Selector  Elements=[2 1 3]  InputPortWidth=3
  Sum : Sum  SaturateOnIntegerOverflow=on
  Sum1 : Sum  Inputs=+-  SaturateOnIntegerOverflow=on
  Sum2 : Sum  Inputs=1  SaturateOnIntegerOverflow=on
  Sum3 : Sum  Inputs=-+  SaturateOnIntegerOverflow=on
  Sum4 : Sum  Inputs=+-  SaturateOnIntegerOverflow=on
  Switch1 : Switch  Threshold=0.5  SaturateOnIntegerOverflow=on
  Trigonometric Function : Trigonometry
  Trigonometric Function1 : Trigonometry  Operator=cos
  Ta_Tb_To : Outport
  wires:
  Odd_S/1 -> Switch1/2
  Switch1/1 -> Ta_Tb_To/1
  Selector1/1 -> Switch1/3
  1/Fc/1 -> Selector1/1, Switch1/1
  Constant/1 -> Sum/2
  Sum4/1 -> Trigonometric Function/1, Sum/1  "alpha1"
  Mux1/1 -> 1/Fc/1
  Sum3/1 -> Mux1/2  "To"
  Product/1 -> Sum2/1, Mux1/1  "TaTb"
  alpha/1 -> Sum4/1
  Product1/1 -> Sum4/2
  Constant2/1 -> Sum1/2
  Sn/1 -> Sum1/1
  Constant1/1 -> Product1/2
  Sum1/1 -> Product1/1
  Constant8/1 -> Sum3/2
  Sum2/1 -> Sum3/1
  Sum/1 -> Trigonometric Function1/1
  m/1 -> Product/1
  Mux/1 -> Product/2
  Trigonometric Function/1 -> Mux/2
  Trigonometric Function1/1 -> Mux/1

== system powerlib_extras/Discrete  Control Blocks/Discrete SV PWM Generator/SV Modulator Pattern #1/Determine the sector of U* based on alpha (rad). Also, determine if the sector number is odd ==
  alpha : Inport  Port=1  LatchInput=off
  Constant1 : Constant  Value=2
  Look-Up Table : Lookup  DialogController=Simulink.DDGSource  InputValues=[0:pi/3:5*pi/3]  OutputValues=[1:6]  SaturateOnIntegerOverflow=on
  Math Function1 : Math  Operator=mod  SaturateOnIntegerOverflow=on
  Rounding Function : Rounding
  Sn : Outport
  Odd_S : Outport  Port=2
  wires:
  alpha/1 -> Look-Up Table/1
  Math Function1/1 -> Odd_S/1
  Constant1/1 -> Math Function1/2
  Rounding Function/1 -> Sn/1, Math Function1/1
  Look-Up Table/1 -> Rounding Function/1

== system powerlib_extras/Discrete  Control Blocks/Discrete SV PWM Generator/SV Modulator Pattern #1/Generate  pulse pattern ==
  note: Column-> pulses for Q1,Q3 et Q5 based on Sector number
  note: Page-> based on which time interval (1 to 7) of the PWM period
  Sn : Inport  Port=1  LatchInput=off
  TaTbTo : Inport  Port=2  LatchInput=off
  Constant2 : Constant
  Constant3 : Constant
  Determine interval of the PWM period based on Ta Tb and To : Subsystem
  Direct Look-Up Table (n-D) : simulink/Lookup Tables/Direct Lookup Table (n-D)  maskTabDims=3  explicitNumDims=1  outDims=Column  tabIsInput=off  mxTable=pat1  clipFlag=Warning
  Logical Operator : Logic  Operator=NOT  AllPortsSameDT=off  OutDataTypeMode=Specify via dialog  LogicDataType=float('double')
  Mux : Mux  Inputs=[3 3]
  Selector : Selector  Elements=[1 4 2 5 3 6]  InputPortWidth=6
  Sum : Sum  Inputs=+-  SaturateOnIntegerOverflow=on
  Sum1 : Sum  Inputs=+-  SaturateOnIntegerOverflow=on
  Pulses : Outport
  wires:
  TaTbTo/1 -> Determine interval of the PWM period based on Ta Tb and To/1(TaTbTo)
  Constant2/1 -> Sum/2
  Sum/1 -> Direct Look-Up Table (n-D)/1  "Page"
  Constant3/1 -> Sum1/2
  Sn/1 -> Sum1/1
  Sum1/1 -> Direct Look-Up Table (n-D)/2  "Column"
  Direct Look-Up Table (n-D)/1 -> Logical Operator/1, Mux/1  "Q1 Q3 Q5"
  Logical Operator/1 -> Mux/2  "Q2 Q4 Q6"
  Mux/1 -> Selector/1
  Selector/1 -> Pulses/1
  Determine interval of the PWM period based on Ta Tb and To/1(Tn) -> Sum/1  "Interval n"

== system powerlib_extras/Discrete  Control Blocks/Discrete SV PWM Generator/SV Modulator Pattern #1/INFO ==
  note: Interval 7
  note: Interval 6
  note: Interval 5
  note: Interval 4
  note: Interval 3
  note: Interval 2
  note: Interval 1
  note: zero
      | space vector
      | (Q1 Q3 Q5 =0)
  note: 1st basic
      | space vector
  note: 2nd basic
      | space vector
  note: zero
      | space vector
      | (Q1 Q3 Q5 =1)
  note: zero
      | space vector
      | (Q1 Q3 Q5 =0)
  note: 2nd basic
      | space vector
  note: 1st basic
      | space vector
  note: Pattern #1 implements the following symmetrical switching pattern:
      | total duration = 1 PWM period (Tpwm = 1/Fc)
  note: |
      | |
      | |
      | |
      | |
      | |
      | |
      | |
      | |
      | |
  note: |
      | |
      | |
      | |
      | |
      | |
      | |
      | |
      | |
      | |
  note: |
      | |
      | |
      | |
      | |
      | |
      | |
      | |
      | |
      | |
  note: |
      | |
      | |
      | |
      | |
      | |
      | |
      | |
      | |
      | |
  note: |
      | |
      | |
      | |
      | |
      | |
      | |
      | |
      | |
      | |
  note: |
      | |
      | |
      | |
      | |
      | |
      | |
      | |
      | |
      | |
  note: Ta/2
  note: To/4
  note: Tb/2
  note: To/2
  note: Tb/2
  note: Ta/2
  note: To/4
  note: Ta=m*cos(alpha+30)* (1/Fc)
  note: Tb=m*sin(alpha) * (1/Fc)
  note: To=(1/Fc-Ta-Tb)
  note: where:
      | Fc = Chopping frequency
      | m = modulation index
      | alpha = angle between reference vector U* and
      | 1st basic space vector

== system powerlib_extras/Discrete  Control Blocks/Discrete SV PWM Generator/SV Modulator Pattern #2/Conv_table ==
  Va : Inport  Port=1  LatchInput=off
  Vb : Inport  Port=2  LatchInput=off
  S : Inport  Port=3  LatchInput=off
  Look-Up Table : Lookup  DialogController=Simulink.DDGSource  InputValues=[1 2 3 4 5 6]  OutputValues=[1 1 0 -1 -1 0]  SaturateOnIntegerOverflow=on
  Look-Up Table1 : Lookup  DialogController=Simulink.DDGSource  InputValues=[1 2 3 4 5 6]  OutputValues=[-1/sqrt(3) 1/sqrt(3) 2/sqrt(3) 1/sqrt(3) -1/sqrt(3) -2/sqrt(3)]  SaturateOnIntegerOverflow=on
  Look-Up Table2 : Lookup  DialogController=Simulink.DDGSource  InputValues=[1 2 3 4 5 6]  OutputValues=[0 -1 -1 0 1 1]  SaturateOnIntegerOverflow=on
  Look-Up Table3 : Lookup  DialogController=Simulink.DDGSource  InputValues=[1 2 3 4 5 6]  OutputValues=[2/sqrt(3) 1/sqrt(3) -1/sqrt(3) -2/sqrt(3) -1/sqrt(3) 1/sqrt(3)]  SaturateOnIntegerOverflow=on
  Product{,1..3} (4 alike) : Product  SaturateOnIntegerOverflow=on  InputSameDT=on
  Sum : Sum  SaturateOnIntegerOverflow=on  InputSameDT=on
  Sum1 : Sum  SaturateOnIntegerOverflow=on  InputSameDT=on
  T1N : Outport
  T2N : Outport  Port=2
  wires:
  S/1 -> Look-Up Table/1, Look-Up Table3/1, Look-Up Table2/1, Look-Up Table1/1
  Va/1 -> Product/1, Product2/1
  Look-Up Table/1 -> Product/2
  Vb/1 -> Product1/1, Product3/1
  Look-Up Table1/1 -> Product1/2
  Look-Up Table2/1 -> Product2/2
  Look-Up Table3/1 -> Product3/2
  Product/1 -> Sum/1
  Product1/1 -> Sum/2
  Product2/1 -> Sum1/1
  Product3/1 -> Sum1/2
  Sum/1 -> T1N/1
  Sum1/1 -> T2N/1

== system powerlib_extras/Discrete  Control Blocks/Discrete Synchronized 12-Pulse Generator/12 Flip-Flops/6 Flip-Flop ==
  S : Inport  Port=1  LatchInput=off
  R : Inport  Port=2  LatchInput=off
  Demux : Demux  Outputs=6
  Demux1 : Demux  Outputs=6
  Mux : Mux  Inputs=6
  S-R Flip-Flop1 : Subsystem  mask(SRFlipFlop){initial_condition=0, Ts=Ts}
      mask prompts: initial_condition "Initial condition:"; Ts "Sample time:"
      mask help: S-R Flip Flop Block
  S-R Flip-Flop2 : Subsystem  mask(SRFlipFlop){initial_condition=0, Ts=Ts}
      mask prompts: initial_condition "Initial condition:"; Ts "Sample time:"
      mask help: S-R Flip Flop Block
  S-R Flip-Flop3 : Subsystem  mask(SRFlipFlop){initial_condition=0, Ts=Ts}
      mask prompts: initial_condition "Initial condition:"; Ts "Sample time:"
      mask help: S-R Flip Flop Block
  S-R Flip-Flop4 : Subsystem  mask(SRFlipFlop){initial_condition=0, Ts=Ts}
      mask prompts: initial_condition "Initial condition:"; Ts "Sample time:"
      mask help: S-R Flip Flop Block
  S-R Flip-Flop5 : Subsystem  mask(SRFlipFlop){initial_condition=0, Ts=Ts}
      mask prompts: initial_condition "Initial condition:"; Ts "Sample time:"
      mask help: S-R Flip Flop Block
  S-R Flip-Flop6 : Subsystem  mask(SRFlipFlop){initial_condition=0, Ts=Ts}
      mask prompts: initial_condition "Initial condition:"; Ts "Sample time:"
      mask help: S-R Flip Flop Block
  Terminator{,1..5} (6 alike) : Terminator
  Q : Outport
  wires:
  S-R Flip-Flop6/2(!Q) -> Terminator5/1
  S-R Flip-Flop5/2(!Q) -> Terminator4/1
  S-R Flip-Flop4/2(!Q) -> Terminator3/1
  S-R Flip-Flop3/2(!Q) -> Terminator2/1
  S-R Flip-Flop2/2(!Q) -> Terminator1/1
  S-R Flip-Flop1/1(Q) -> Mux/1
  S-R Flip-Flop2/1(Q) -> Mux/2
  S-R Flip-Flop3/1(Q) -> Mux/3
  S-R Flip-Flop4/1(Q) -> Mux/4
  S-R Flip-Flop5/1(Q) -> Mux/5
  Mux/1 -> Q/1
  S-R Flip-Flop6/1(Q) -> Mux/6
  S-R Flip-Flop1/2(!Q) -> Terminator/1
  Demux/1 -> S-R Flip-Flop1/1(S)
  Demux/2 -> S-R Flip-Flop2/1(S)
  Demux/3 -> S-R Flip-Flop3/1(S)
  Demux/4 -> S-R Flip-Flop4/1(S)
  S/1 -> Demux/1
  Demux/6 -> S-R Flip-Flop6/1(S)
  Demux/5 -> S-R Flip-Flop5/1(S)
  R/1 -> Demux1/1
  Demux1/1 -> S-R Flip-Flop1/2(R)
  Demux1/2 -> S-R Flip-Flop2/2(R)
  Demux1/3 -> S-R Flip-Flop3/2(R)
  Demux1/4 -> S-R Flip-Flop4/2(R)
  Demux1/5 -> S-R Flip-Flop5/2(R)
  Demux1/6 -> S-R Flip-Flop6/2(R)
